simulink subsystem "SubSystemMotorConveyor"  (R2020b)
settings: Solver=VariableStepAuto  StartTime=0.0  StopTime=10.0  RelTol=1e-3
settings Model: Creator=kaebi  LastModifiedBy=kaebi

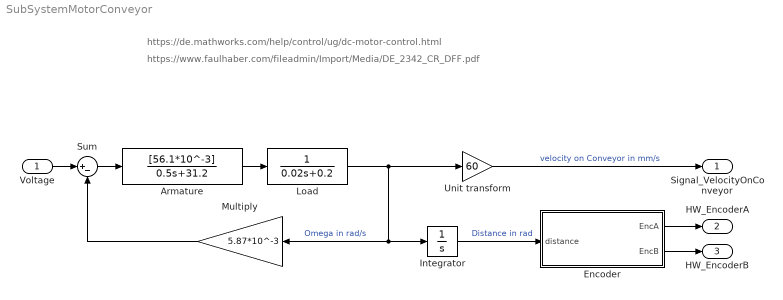
== system SubSystemMotorConveyor ==
  note: https://de.mathworks.com/help/control/ug/dc-motor-control.html
  note: https://www.faulhaber.com/fileadmin/Import/Media/DE_2342_CR_DFF.pdf
  Voltage : Inport
  Armature : TransferFcn  Numerator=[56.1*10^-3]  Denominator=[0.5 31.2]
  Encoder : MATLAB Function  TreatAsAtomicUnit=on
  Integrator : Integrator
  Load : TransferFcn  Denominator=[0.02 0.2]
  Multiply : Gain  Gain=5.87*10^-3
  Sum : Sum  Inputs=|+-
  Unit transform : Gain  Gain=60
  Signal_VelocityOnConveyor : Outport
  HW_EncoderA : Outport  Port=2
  HW_EncoderB : Outport  Port=3
  wires:
  Encoder/2(EncB) -> HW_EncoderB/1
  Encoder/1(EncA) -> HW_EncoderA/1
  Integrator/1 -> Encoder/1(distance)  "Distance in rad"
  Unit transform/1 -> Signal_VelocityOnConveyor/1  "velocity on Conveyor in mm/s"
  Multiply/1 -> Sum/2
  Voltage/1 -> Sum/1
  Sum/1 -> Armature/1
  Load/1 -> Unit transform/1, Multiply/1, Integrator/1  "Omega in rad/s"
  Armature/1 -> Load/1

== matlab function SubSystemMotorConveyor/Encoder ==
  data: distance input; EncA output; EncB output
function [EncA, EncB] = fcn(distance)
    impulseDistance = 2*pi/1024;
    
    currentDistA = mod(distance, impulseDistance);
    currentDistB = mod(distance+(impulseDistance*0.25), impulseDistance);
    
    if (currentDistA < impulseDistance*0.5)
        EncA = 1;
    else
        EncA = 0;
    end
    
    if (currentDistB < impulseDistance*0.5)
        EncB = 1;
    else
        EncB = 0;
    end
end
